simulink model "sim_ukf_est_motor_4para_variable_load"  (R2020b)
settings: Solver=ode1  StartTime=0.0  StopTime=300  FixedStep=0.01  RelTol=1e-3
settings Model: Creator=Admin  LastModifiedBy=ONLY-GOD

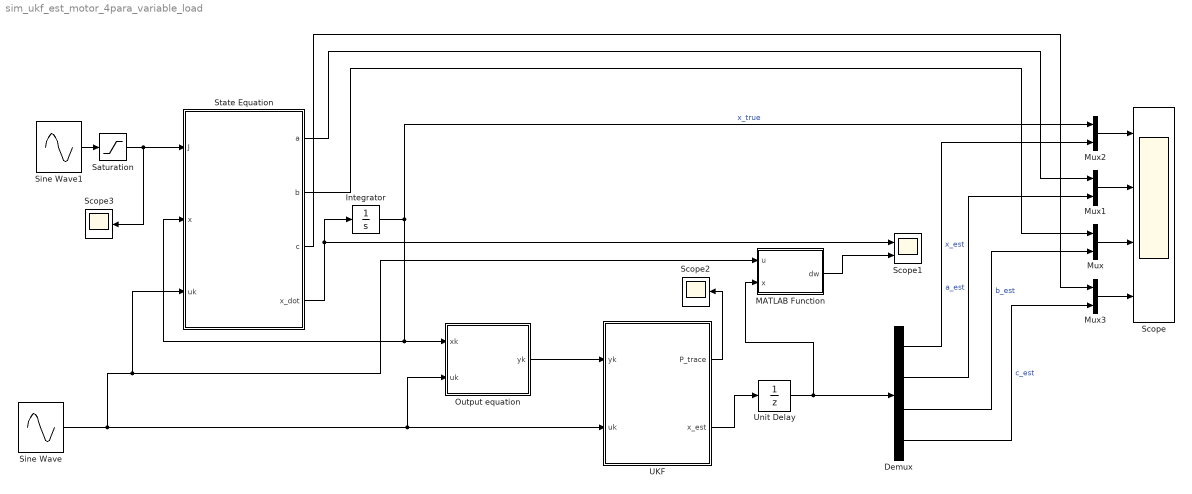
== system sim_ukf_est_motor_4para_variable_load ==
  Demux : Demux
  Integrator : Integrator
  MATLAB Function : MATLAB Function  TreatAsAtomicUnit=on
  Mux{,1..3} (4 alike) : Mux  Inputs=2
  Output equation : MATLAB Function  TreatAsAtomicUnit=on
  Saturation : Saturate  UpperLimit=1.94e-4*0.05*0.4  LowerLimit=1.94e-4*0.05*0.1
  Scope : Scope  NumInputPorts=4
  Scope1 : Scope  NumInputPorts=2
  Scope2 : Scope
  Scope3 : Scope
  Sine Wave : Sin  Amplitude=5  Bias=5  Frequency=2*pi/20  SampleTime=0
  Sine Wave1 : Sin  Amplitude=1.94e-4*0.05*0.5  Bias=1.94e-4*0.05*0.5  Frequency=2*pi/100  SampleTime=0
  State Equation : MATLAB Function  TreatAsAtomicUnit=on
  UKF : MATLAB Function  TreatAsAtomicUnit=on
  Unit Delay : UnitDelay  InitialCondition=[0;0;0;0]  SampleTime=-1  HasFrameUpgradeWarning=on
  wires:
  Integrator/1 -> Mux2/1, State Equation/2(x), Output equation/1(xk)  "x_true"
  Sine Wave/1 -> State Equation/3(uk), MATLAB Function/1(u), Output equation/2(uk), UKF/2(uk)
  State Equation/4(x_dot) -> Integrator/1, Scope1/1
  Output equation/1(yk) -> UKF/1(yk)
  Unit Delay/1 -> MATLAB Function/2(x), Demux/1
  Mux2/1 -> Scope/1
  Mux1/1 -> Scope/2
  Mux/1 -> Scope/3
  Mux3/1 -> Scope/4
  Demux/4 -> Mux3/2  "c_est"
  Demux/3 -> Mux/2  "b_est"
  Demux/2 -> Mux1/2  "a_est"
  Demux/1 -> Mux2/2  "x_est"
  MATLAB Function/1(dw) -> Scope1/2
  UKF/2(x_est) -> Unit Delay/1
  UKF/1(P_trace) -> Scope2/1
  Sine Wave1/1 -> Saturation/1
  State Equation/1(a) -> Mux1/1
  State Equation/2(b) -> Mux/1
  State Equation/3(c) -> Mux3/1
  Saturation/1 -> Scope3/1, State Equation/1(J)

== matlab function sim_ukf_est_motor_4para_variable_load/MATLAB Function ==
  data: u input; dw output; x input
function dw = fcn(u,x)

dw = -x(2)*x(1)+x(3)*u-x(4)*sign(x(1));

== matlab function sim_ukf_est_motor_4para_variable_load/State Equation ==
  settings: updateMethod=DISCRETE
  data: a output; b output; c output; J input; x input; uk input; x_dot output
function [a,b,c,x_dot] = state_eq(J,x,uk)
% x1 = W , x2 = a , x3 = b , x4 = c

Ra = 14.3;
Kt = 0.05;
Kb = 0.063;
Tc = 0.053*Kt;
D  = 9.4e-5*Kt;
J0 = 1.94e-4*Kt + J;

a = (Kt*Kb+Ra*D)/Ra/J0;
b = Kt/Ra/J0;
c = Tc/J0;
x_dot = -a*x + b*uk - c*sign(x);

== matlab function sim_ukf_est_motor_4para_variable_load/Output equation ==
  data: yk output size=[1,1]; xk input; uk input
function yk = fcn(xk,uk)

y_tem = hd(uk,xk);
yk = y_tem(1:1,1);
end

% Customized function

function y = hd(~,x)
C = [1,0,0,0];
y = C*x;
end

== matlab function sim_ukf_est_motor_4para_variable_load/UKF ==
  settings: updateMethod=DISCRETE
  data: P_trace output; x_est output; yk input size=[1,1]; uk input
function [P_trace,x_est] = fcn(yk,uk)
Ts = 0.01;
Qc = 1e-1*diag([0.1;0.1;15;10]);
R = 2e-5;
persistent n m xk1 Pk1 wm W lambda nsigma
n = 4; % number of state
m = 1; % number of output

if isempty(xk1)
    xk1= randn(n,1); Pk1 = 1e-1*eye(n);
    nsigma = 2*n+1; k=2;
    alpha=0.5; beta=1;
    lambda=alpha^2*(n+k)-n;
    Wm0=lambda/(n+lambda);
    Wc0=lambda/((n+lambda)+(1-alpha^2+beta));
    Wmi=1/2/(n+lambda);
    Wci=Wmi;
    wm=Wmi*ones(nsigma,1); wm(1)=Wm0;
    W=(eye(nsigma)-wm*ones(1,nsigma))...
     *diag([Wc0 Wci*ones(1,2*n)])...
     *(eye(nsigma)-wm*ones(1,nsigma))';
end
tic
%Measurement Update
%Generate Sigma Points
x = xk1; P = Pk1;
A   = chol(P,'lower');
X   = x*ones(1,nsigma) + ...
        sqrt(n+lambda)*[zeros(n,1) A -A];
Y   = zeros(m,nsigma);
for i=1:nsigma
    Y(:,i)= hd(uk,X(:,i));
end
y   = Y*wm;
Pxy = X*W*Y';
Pyy = Y*W*Y'+R;
K   = Pxy/Pyy;
x   = x + K*(yk-y);
P   = P - K*Pyy*K';

%Time Update
%Generate Sigma Points
A = chol(P,'lower');
X = x*ones(1,nsigma) + ...
        sqrt(n+lambda)*[zeros(n,1) A -A];
Xk1 = zeros(n,nsigma);
for i=1:nsigma
    Xk1(:,i)= fd(uk,X(:,i),Ts);
end
xk1     = Xk1*wm;
Pk1     = Xk1*W*Xk1'+Qc*Ts;
x_est   = xk1(1:4,1);
P_trace = trace(Pk1);
toc
end

function y = hd(~,x)
C = [1,0,0,0];
y = C*x;
end

% Customizable function fc for various equation
function xk1 = fd(u,x,Ts)

% Continuous function
% function x_dot = fc(u,x)
% theta_ddot = -a*theta_do + b*u
% Let x(1)=theta_dot, x(2)=a, x(3)=b, x(4)=c, then
% x_dot(1) = x(2)
% x_dot(2) = -x(3)*x(2) + x(4)*u
% x_dot(3) = 0    (since a is constant)
% x_dot(4) = 0    (since b is constant)
% In compact form
% x_dot = fc(u,x)
x_dot = zeros(4,1);
x_dot(1,1) = -x(1,1)*x(2,1) + x(3,1)*u-x(4,1)*sign(x(1,1));
x_dot(2,1) = 0;
x_dot(3,1) = 0;
x_dot(4,1) = 0;
% end

% Discretization
xk1 = x + x_dot*Ts;
end
